simulink model "app"  (R2023b)
settings: Solver=FixedStepDiscrete  StartTime=0.0  StopTime=10.0  FixedStep=0.001  RelTol=1e-3  EnableMultiTasking=on
libraries: ncukit x6
settings Model: SimulationMode=external  Creator=sebam  LastModifiedBy=sebam
settings OptimizationCC: DefaultParameterBehavior=Inlined  EnhancedBackFolding=on  PassReuseOutputArgsAs=Individual arguments  ZeroExternalMemoryAtStartup=off  ZeroInternalMemoryAtStartup=off  MaxStackSize=64  OptimizeBlockOrder=speed  DifferentSizesBufferReuse=on  OptimizationCustomize=off  EfficientTunableParamExpr=on
settings DebuggingCC: ParameterTunabilityLossMsg=error
settings HardwareCC: ProdBitPerPointer=32  ProdBitPerSizeT=32  ProdBitPerPtrDiffT=32  ProdLargestAtomicInteger=Long  ProdLargestAtomicFloat=Double  ProdWordSize=32  ProdHWDeviceType=NCU->ARM Cortex-M
settings SFSimCC: MATLABDynamicMemAlloc=off
settings RTWCC: Description=NCU Networking ECU  SystemTargetFile=ncu.tlc  HardwareBoard=NCU  TemplateMakefile=ert_default_tmf  PostCodeGenCommand=ncu_build_hook  Toolchain=NCU STM32 CMake  BuildConfiguration=Release
settings CodeAppCC: ForceParamTrailComments=on  IgnoreCustomStorageClasses=off  OperatorAnnotations=on  SimulinkDataObjDesc=on  SFDataObjDesc=on  InsertBlockDesc=on
settings STFCustomTargetCC: TargetLangStandard=C89/C90 (ANSI)  MultiwordLength=256  ModelReferenceCompliant=off  CombineOutputUpdateFcns=on  ERTCustomFileBanners=on  SupportContinuousTime=off  SupportNonInlinedSFcns=off  RemoveResetFunc=on  MATLABClassNameForMDSCustomization=Simulink.SoftwareTarget.ERTCustomization  UseToolchainInfoCompliant=on  SystemTargetFile=ncu.tlc
settings ERTTargetCC: ModelReferenceCompliant=off  ParMdlRefBuildCompliant=off  CompOptLevelCompliant=off  ConcurrentExecutionCompliant=off  ModelStepFunctionPrototypeControlCompliant=off  CPPClassGenCompliant=off  InlinedParameterPlacement=NonHierarchical  ERTCustomFileTemplate=example_file_process.tlc

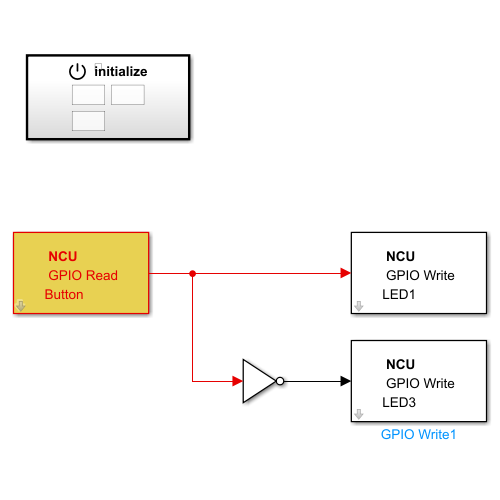
[thumbnail: Simulink's stored preview of the top-level diagram]
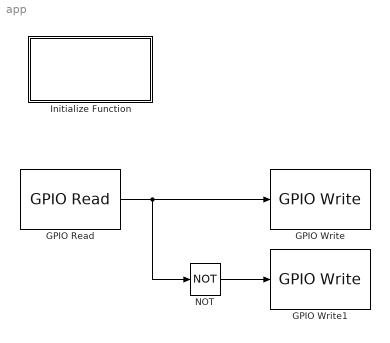
== system app ==
  GPIO Read : ncukit/GPIO/GPIO Read  pin=gpio_pin.Button
  GPIO Write : ncukit/GPIO/GPIO Write  pin=gpio_pin.LED1
  GPIO Write1 : ncukit/GPIO/GPIO Write  pin=gpio_pin.LED3
  Initialize Function : Subsystem  TreatAsAtomicUnit=on
  NOT : Logic  Operator=NOT  IconShape=distinctive  AllPortsSameDT=off  OutDataTypeStr=boolean
  wires:
  GPIO Read/1 -> NOT/1, GPIO Write/1
  NOT/1 -> GPIO Write1/1

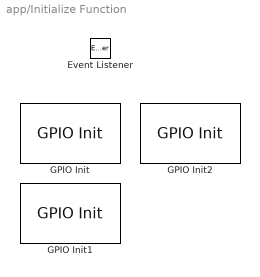
== system app/Initialize Function ==
  Event Listener : EventListener  DisableCoverage=on  EventName=reset
  GPIO Init : ncukit/GPIO/GPIO Init  pin=gpio_pin.LED1  isInput=Output
  GPIO Init1 : ncukit/GPIO/GPIO Init  pin=gpio_pin.Button  isInput=Input
  GPIO Init2 : ncukit/GPIO/GPIO Init  pin=gpio_pin.LED3  isInput=Output
